simulink model "SerialWriteTriggeredSubsystem_v2"  (R2018a)
settings: Solver=FixedStepAuto  StartTime=0.0  StopTime=inf  FixedStep=.01  RelTol=1e-3  EnableMultiTasking=on
libraries: arduinolib x3, ArduinoCustomLibrary x1, simulink x1
settings Model: ExtModeTrigDuration=2  Creator=jonathancoulter  LastModifiedBy=jonathancoulter
settings SolverCC: AutoInsertRateTranBlk=on
settings OptimizationCC: EnhancedBackFolding=on  PassReuseOutputArgsAs=Individual arguments  MaxStackSize=64  OptimizeBlockOrder=speed  DifferentSizesBufferReuse=on  OptimizationCustomize=off
settings DebuggingCC: ParameterTunabilityLossMsg=error
settings HardwareCC: ProdBitPerInt=16  ProdBitPerPointer=16  ProdBitPerSizeT=16  ProdBitPerPtrDiffT=16  ProdLargestAtomicFloat=None  ProdWordSize=8  ProdHWDeviceType=Atmel->AVR  UseEmbeddedCoderFeatures=off
settings SFSimCC: MATLABDynamicMemAlloc=off
settings RTWCC: SystemTargetFile=ert.tlc  HardwareBoard=Arduino Mega 2560  TLCOptions=-aInlineSetEventsForThisBaseRateFcn=TLC_FALSE -aSuppressMultiTaskScheduler=TLC_FALSE -aRateBasedStepFcn=1  TemplateMakefile=ert_default_tmf  Toolchain=Arduino AVR  BuildConfiguration=Faster Runs  IncludeHyperlinkInReport=on
settings CodeAppCC: ForceParamTrailComments=on  IgnoreCustomStorageClasses=off  OperatorAnnotations=on  SimulinkDataObjDesc=on  SFDataObjDesc=on  InsertBlockDesc=on
settings ERTTargetCC: SupportContinuousTime=on  SupportNonInlinedSFcns=on  SupportVariableSizeSignals=on

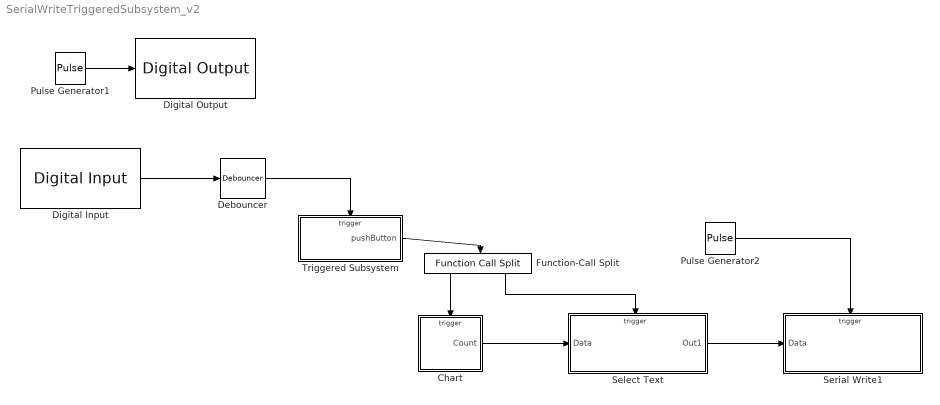
== system SerialWriteTriggeredSubsystem_v2 ==
  Chart : Stateflow chart  TreatAsAtomicUnit=on
  Debouncer : ArduinoCustomLibrary/Debouncer
      settings: SourceProductName=Custom Arduino
  Digital Input : arduinolib/Digital Input  pinNumber=8  sampleTime=.05  blockPlatform=arduino
      settings: SourceProductName=Simulink Support Package for Arduino Hardware
  Digital Output : arduinolib/Digital Output  pinNumber=13  blockPlatform=arduino
  Function-Call Split : FunctionCallSplit  IconShape=distinctive  NumOutputPorts=2  OutputPortLayout=default
  Pulse Generator1 : DiscretePulseGenerator  SampleTime=-1
  Pulse Generator2 : DiscretePulseGenerator  PulseType=Time based  Period=1  PulseWidth=50  SampleTime=-1
  Select Text : Subsystem
  Serial Write1 : Subsystem
  Triggered Subsystem : Subsystem  TreatAsAtomicUnit=on
  wires:
  Pulse Generator1/1 -> Digital Output/1
  Digital Input/1 -> Debouncer/1
  Debouncer/1 -> Triggered Subsystem/Trigger
  Chart/1(Count) -> Select Text/1(Data)
  Select Text/1(Out1) -> Serial Write1/1(Data)
  Triggered Subsystem/1(pushButton) -> Function-Call Split/1
  Pulse Generator2/1 -> Serial Write1/Trigger
  Function-Call Split/1 -> Chart/Trigger
  Function-Call Split/2 -> Select Text/Trigger

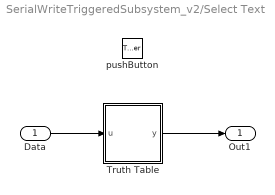
== system SerialWriteTriggeredSubsystem_v2/Select Text ==
  Data : Inport
  pushButton : TriggerPort  TriggerType=function-call  VariantControl=Variant  PortDimensions=1
  Truth Table : Truth Table  TreatAsAtomicUnit=on
  Out1 : Outport
  wires:
  Data/1 -> Truth Table/1(u)
  Truth Table/1(y) -> Out1/1

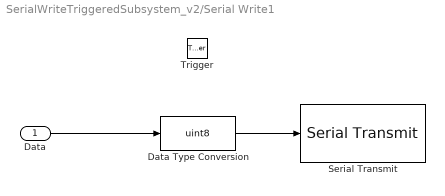
== system SerialWriteTriggeredSubsystem_v2/Serial Write1 ==
  Data : Inport
  Trigger : TriggerPort  VariantControl=Variant  PortDimensions=1
  Data Type Conversion : DataTypeConversion  OutDataTypeStr=uint8
  Serial Transmit : arduinolib/Serial Transmit  portNumber=0  sendmode=write  sendformat=Decimal  floatprecision=2  blockPlatform=arduino
      settings: SourceProductName=Simulink Support Package for Arduino Hardware
  wires:
  Data Type Conversion/1 -> Serial Transmit/1
  Data/1 -> Data Type Conversion/1

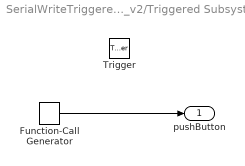
== system SerialWriteTriggeredSubsystem_v2/Triggered Subsystem ==
  Trigger : TriggerPort  VariantControl=Variant
  Function-Call Generator : simulink/Ports & Subsystems/Function-Call Generator  sample_time=-1  numberOfIterations=1
  pushButton : Outport
  wires:
  Function-Call Generator/1 -> pushButton/1

== matlab function SerialWriteTriggeredSubsystem_v2/Select Text/Truth Table ==
  data: u input; y output
function y = fcn(u)

aVarTruthTableCondition_1 = false;
aVarTruthTableCondition_2 = false;
aVarTruthTableCondition_3 = false;


% Text 1

aVarTruthTableCondition_1 = logical(u == 1);

% Text 2

aVarTruthTableCondition_2 = logical(u == 2);

% Text 3

aVarTruthTableCondition_3 = logical(u == 3);

if (aVarTruthTableCondition_1 && ~aVarTruthTableCondition_2 && ~aVarTruthTableCondition_3)
    aFcnTruthTableAction_1();
elseif (~aVarTruthTableCondition_1 && aVarTruthTableCondition_2 && ~aVarTruthTableCondition_3)
    aFcnTruthTableAction_2();
elseif (~aVarTruthTableCondition_1 && ~aVarTruthTableCondition_2 && aVarTruthTableCondition_3)
    aFcnTruthTableAction_3();
else % Default
    aFcnTruthTableAction_4();
end

function aFcnTruthTableAction_1()

% Text 1

y = [abs('First text '), 10]';

function aFcnTruthTableAction_2()

% Text 2

y = [abs('Second text'), 10]';

function aFcnTruthTableAction_3()

% Text 3

y = [abs('Third text '), 10]';

function aFcnTruthTableAction_4()

% Error

y = [abs('Error      '), 10]';

== stateflow chart SerialWriteTriggeredSubsystem_v2/Chart ==
  settings: executeAtInitialization=1
  state Init
  (default) -> Init : {Count = 1;}
  Init -> Init [order 2] : [Count == 3]{Count = 1;}
  Init -> Init [order 1] : [Count < 3]{Count = Count + 1}
  data: Count output uint8 =uint8(1)
  events: pushButton input FUNCTION_CALL_EVENT
